simulink model "A"  (R2024b)
settings: Solver=VariableStepAuto  StartTime=0.0  StopTime=0.5  RelTol=1e-3
undefined symbols (not defined in the file): Ion, Lithium
libraries: spsSeriesRLCBranchLib x11, spsVoltageMeasurementLib x7, spsMosfetLib x6, spsCurrentMeasurementLib x4, spsPVArrayLib x2, spsDiodeLib x2, spsBatteryLib x2, slpidlib x2, spsTriangleGeneratorLib x2, spsBreakerLib x1, spspowerguiLib x1
settings Model: Creator=ASUS  LastModifiedBy=ASUS

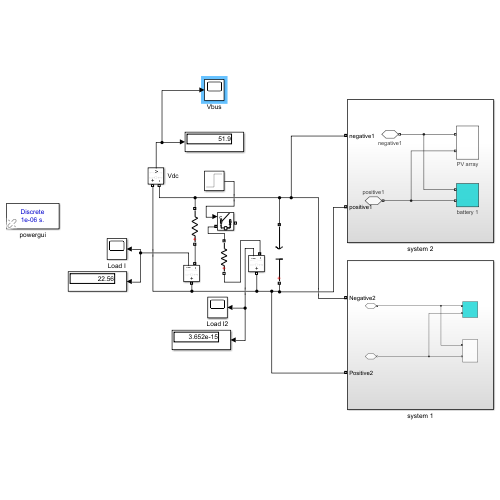
[thumbnail: Simulink's stored preview of the top-level diagram]
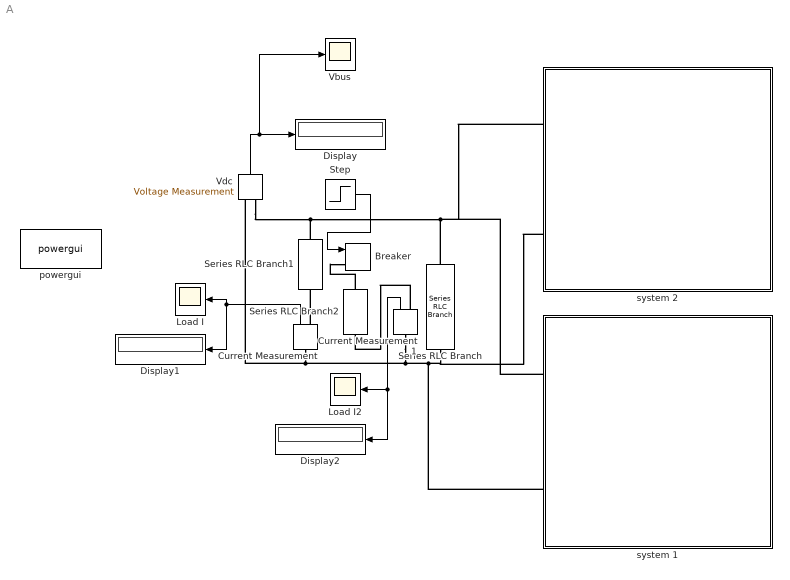
== system A ==
  Breaker : spsBreakerLib/Breaker  InitialState=0  SwitchingTimes="[1/60  5/60]"  External=on  BreakerResistance=0.01  SnubberResistance=1e6  SnubberCapacitance=inf  Measurements=None  MoreParameters=on  NoBreakLoop=off
  Current Measurement : spsCurrentMeasurementLib/Current Measurement  PhasorSimulation=off  OutputType=Complex  PSBequivalent=0
  Current Measurement1 : spsCurrentMeasurementLib/Current Measurement  PhasorSimulation=off  OutputType=Complex  PSBequivalent=0
  Display : Display
  Display1 : Display
  Display2 : Display
  Load I : Scope
  Load I2 : Scope
  Series RLC Branch : spsSeriesRLCBranchLib/Series RLC Branch  LConnTagsString=__new0  RConnTagsString=__new0  BranchType=C  Resistance=1  Inductance=1e-3  SetiL0=off  InitialCurrent=0  Capacitance=4700e-6  Setx0=off  InitialVoltage=0  Measurements=None
  Series RLC Branch1 : spsSeriesRLCBranchLib/Series RLC Branch  LConnTagsString=__new0  RConnTagsString=__new0  BranchType=R  Resistance=2.3  Inductance=1e-3  SetiL0=off  InitialCurrent=0  Capacitance=4700e-6  Setx0=off  InitialVoltage=0  Measurements=None
  Series RLC Branch2 : spsSeriesRLCBranchLib/Series RLC Branch  LConnTagsString=__new0  RConnTagsString=__new0  BranchType=R  Resistance=2.3  Inductance=1e-3  SetiL0=off  InitialCurrent=0  Capacitance=4700e-6  Setx0=off  InitialVoltage=0  Measurements=None
  Step : Step  Time=0.2  SampleTime=0
  Vbus : Scope
  Vdc : spsVoltageMeasurementLib/Voltage Measurement  PhasorSimulation=off  OutputType=Complex  PSBequivalent=0
  powergui : spspowerguiLib/powergui  Priority=1  SimulationMode=Discrete  SampleTime=1e-6  frequency=60  Iterations=50  frequencyindice=0  Pbase=100e6  ErrMax=1e-4  UnitsV=kV  UnitsW=MW  buscounter=0  FunctionMessages=off  echomessages=off  EnableUseOfTLC=off  CurrentSourceSwitches=off  DisableSnubberDevices=off  DisableRonSwitches=off  DisableVfSwitches=off  DisplayEquations=off  AutomaticDiscreteSolvers=off  SolverType=Tustin/Backward Euler (TBE)  Interpol=off  ExternalGateDelay=off  methode=off  Ts=100  x0status=blocks  SPID=on  SwTol=0  HookPort=off  NonlinearTolerance=1e-4  nMaxIteration=100  ContinueOnMaxIteration=off  RestoreLinks=warning  ResistiveCurrentMeasurement=off  Frange=[0:2:500]  Ylog=off  Xlog=on  ShowGrid=off  save=off  variable=ZData  structure=0  ZoomFFT=off  StartTime=0.0  cycles=1  DisplayStyle=1  fundamental=60  FreqAxis=off  MaxFrequency=1000  frequencyindicesteady=1  RmsSteady=1  display=off
  system 1 : Subsystem
  system 2 : Subsystem
  wires:
  Vdc/1 -> Vbus/1, Display/1
  Step/1 -> Breaker/1
  Current Measurement/1 -> Load I/1, Display1/1
  Current Measurement1/1 -> Display2/1, Load I2/1
  connections:
  system 2/LConn2 -- Series RLC Branch/LConn1 -- system 1/LConn2 -- Current Measurement1/LConn1 -- Current Measurement/LConn1 -- Vdc/LConn1
  Vdc/LConn2 -- Series RLC Branch1/RConn1 -- system 2/LConn1 -- system 1/LConn1 -- Series RLC Branch/RConn1
  Series RLC Branch2/RConn1 -- Breaker/LConn1
  Current Measurement/RConn1 -- Series RLC Branch1/LConn1
  Current Measurement1/RConn1 -- Series RLC Branch2/LConn1

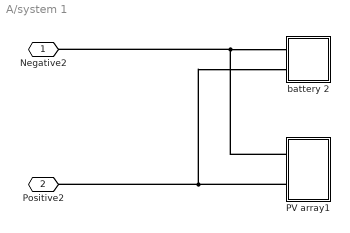
== system A/system 1 ==
  PV array1 : Subsystem
  battery 2 : Subsystem
  Negative2 : PMIOPort  Side=Left
  Positive2 : PMIOPort  Port=2  Side=Left
  connections:
  PV array1/LConn2 -- Positive2/RConn1 -- battery 2/LConn2
  PV array1/LConn1 -- Negative2/RConn1 -- battery 2/LConn1

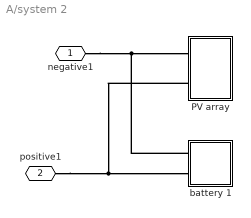
== system A/system 2 ==
  PV array : Subsystem
  battery 1 : Subsystem
  negative1 : PMIOPort  Side=Left
  positive1 : PMIOPort  Port=2  Side=Left
  connections:
  PV array/LConn2 -- positive1/RConn1 -- battery 1/LConn2
  battery 1/LConn1 -- negative1/RConn1 -- PV array/LConn1

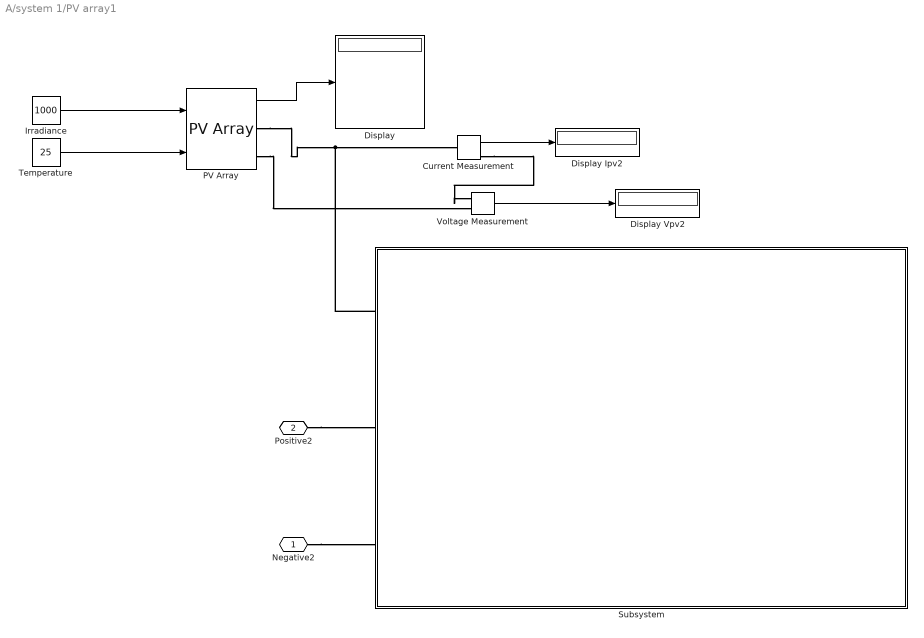
== system A/system 1/PV array1 ==
  Current Measurement : spsCurrentMeasurementLib/Current Measurement  PhasorSimulation=off  OutputType=Complex  PSBequivalent=0
  Display : Display
  Display Ipv2 : Display
  Display Vpv2 : Display
  Irradiance : Constant  Value=1000
  PV Array : spsPVArrayLib/PV Array  Npar=5  Nser=1  PlotType=array @ 1000 W/m2 & specified temperatures  S_vec="[ 1000  500  100 ]"  Temp_C_vec="[ 45 25  ]"  ModuleName=Kyocera Solar KC200GT  PlotWhenSelected=off  Pm=200.143  Ncell=54  Voc=32.9  Isc=8.21  Vm=26.3  Im=7.61  beta_Voc_pc=-0.355  alpha_Isc_pc=0.06  beta_Voc=-0.11679  alpha_Isc=0.004926  IL=8.2288  I0=2.3234e-10  nI=0.97734  Rsh=150.6844  Rs=0.34484  RobustModel=off  RobustCellTemperature=313.3991  BAL=off  Tc=1e-6  Tfilter=5e-5
  Subsystem : Subsystem
  Temperature : Constant  Value=25
  Voltage Measurement : spsVoltageMeasurementLib/Voltage Measurement  PhasorSimulation=off  OutputType=Complex  PSBequivalent=0
  Negative2 : PMIOPort  Side=Left
  Positive2 : PMIOPort  Port=2  Side=Left
  wires:
  Current Measurement/1 -> Display Ipv2/1
  Irradiance/1 -> PV Array/1
  Voltage Measurement/1 -> Display Vpv2/1
  PV Array/1 -> Display/1
  Temperature/1 -> PV Array/2
  connections:
  PV Array/RConn1 -- Subsystem/LConn1 -- Current Measurement/LConn1
  PV Array/RConn2 -- Voltage Measurement/LConn2
  Current Measurement/RConn1 -- Voltage Measurement/LConn1
  Negative2/RConn1 -- Subsystem/LConn3
  Positive2/RConn1 -- Subsystem/LConn2

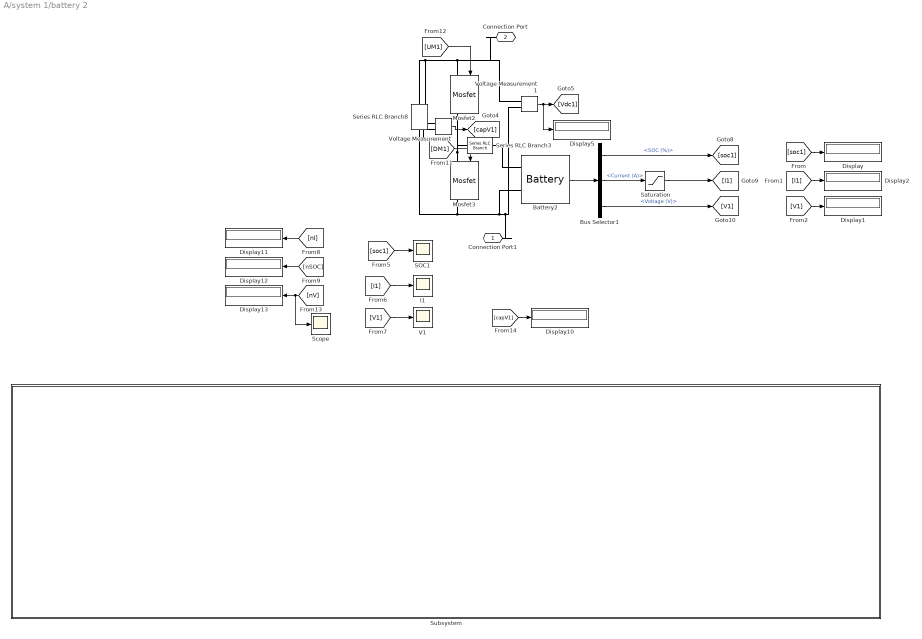
== system A/system 1/battery 2 ==
  Battery2 : spsBatteryLib/Battery  BatType=Lithium-Ion  NomV=50  NomQ=5  SOC=60  Batt_Tr=30  PresetModel=on  MaxQ=5  MinV=37.5  FullV=58.1994  Dis_rate=2.1739  R=0.1  Normal_OP=4.5217  expZone="[54.0193     0.245652]"
  Bus Selector1 : BusSelector  OutputSignals=SOC (%),Current (A),Voltage (V)
  Display{,1..2,5,10..13} (8 alike) : Display
  I1 : Scope
  Mosfet2 : spsMosfetLib/Mosfet  Ron=0.1  Lon=0  Rd=0.01  Vfd=0  IC=0  Rs=1e6  Cs=inf  Measurements=on
  Mosfet3 : spsMosfetLib/Mosfet  Ron=0.1  Lon=0  Rd=0.01  Vfd=0  IC=0  Rs=1e6  Cs=inf  Measurements=on
  SOC1 : Scope
  Saturation : Saturate  UpperLimit=31.5  LowerLimit=-31.5
  Scope : Scope
  Series RLC Branch3 : spsSeriesRLCBranchLib/Series RLC Branch  LConnTagsString=__new0  RConnTagsString=__new0  BranchType=L  Resistance=1  Inductance=500e-6  SetiL0=off  InitialCurrent=0  Capacitance=1e-6  Setx0=off  InitialVoltage=0  Measurements=None
  Series RLC Branch8 : spsSeriesRLCBranchLib/Series RLC Branch  LConnTagsString=__new0  RConnTagsString=__new0  BranchType=RC  Resistance=1  Inductance=1e-3  SetiL0=off  InitialCurrent=0  Capacitance=1500e-6  Setx0=off  InitialVoltage=0  Measurements=None
  Subsystem : Subsystem
  V1 : Scope
  Voltage Measurement : spsVoltageMeasurementLib/Voltage Measurement  PhasorSimulation=off  OutputType=Complex  PSBequivalent=0
  Voltage Measurement1 : spsVoltageMeasurementLib/Voltage Measurement  PhasorSimulation=off  OutputType=Complex  PSBequivalent=0
  Connection Port1 : PMIOPort  Side=Left
  Connection Port : PMIOPort  Port=2  Side=Left
  wires:
  [soc1] -> Display/1
  Voltage Measurement/1 -> [capV1]
  [nSOC] -> Display12/1
  [V1] -> V1/1
  [nI] -> Display11/1
  Bus Selector1/3 -> [V1]  "<Voltage (V)>"
  [UM1] -> Mosfet2/1
  Battery2/1 -> Bus Selector1/1
  [I1] -> Display2/1
  [soc1] -> SOC1/1
  [nV] -> Display13/1, Scope/1
  Bus Selector1/1 -> [soc1]  "<SOC (%)>"
  [I1] -> I1/1
  [capV1] -> Display10/1
  [V1] -> Display1/1
  [DM1] -> Mosfet3/1
  Voltage Measurement1/1 -> [Vdc1], Display5/1
  Saturation/1 -> [I1]
  Bus Selector1/2 -> Saturation/1  "<Current (A)>"
  connections:
  Mosfet3/LConn1 -- Series RLC Branch3/RConn1 -- Mosfet2/RConn1
  Voltage Measurement1/LConn2 -- Connection Port1/RConn1 -- Mosfet3/RConn1 -- Voltage Measurement/LConn2 -- Series RLC Branch8/RConn1 -- Battery2/LConn2
  Voltage Measurement/LConn1 -- Connection Port/RConn1 -- Voltage Measurement1/LConn1 -- Mosfet2/LConn1 -- Series RLC Branch8/LConn1
  Battery2/LConn1 -- Series RLC Branch3/LConn1

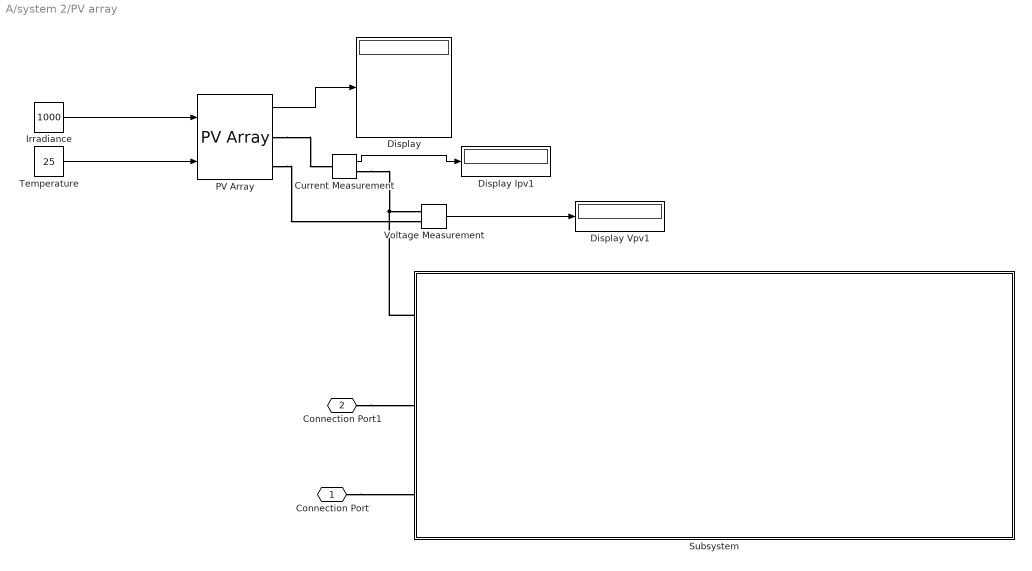
== system A/system 2/PV array ==
  Current Measurement : spsCurrentMeasurementLib/Current Measurement  PhasorSimulation=off  OutputType=Complex  PSBequivalent=0
  Display : Display
  Display Ipv1 : Display
  Display Vpv1 : Display
  Irradiance : Constant  Value=1000
  PV Array : spsPVArrayLib/PV Array  Npar=5  Nser=1  PlotType=array @ 1000 W/m2 & specified temperatures  S_vec="[ 1000  500  100 ]"  Temp_C_vec="[ 45 25  ]"  ModuleName=Kyocera Solar KC200GT  PlotWhenSelected=off  Pm=200.143  Ncell=54  Voc=32.9  Isc=8.21  Vm=26.3  Im=7.61  beta_Voc_pc=-0.355  alpha_Isc_pc=0.06  beta_Voc=-0.11679  alpha_Isc=0.004926  IL=8.2288  I0=2.3234e-10  nI=0.97734  Rsh=150.6844  Rs=0.34484  RobustModel=off  RobustCellTemperature=313.3991  BAL=off  Tc=1e-6  Tfilter=5e-5
  Subsystem : Subsystem
  Temperature : Constant  Value=25
  Voltage Measurement : spsVoltageMeasurementLib/Voltage Measurement  PhasorSimulation=off  OutputType=Complex  PSBequivalent=0
  Connection Port : PMIOPort  Side=Left
  Connection Port1 : PMIOPort  Port=2  Side=Left
  wires:
  Temperature/1 -> PV Array/2
  PV Array/1 -> Display/1
  Voltage Measurement/1 -> Display Vpv1/1
  Irradiance/1 -> PV Array/1
  Current Measurement/1 -> Display Ipv1/1
  connections:
  Current Measurement/RConn1 -- Subsystem/LConn1 -- Voltage Measurement/LConn1
  PV Array/RConn2 -- Voltage Measurement/LConn2
  PV Array/RConn1 -- Current Measurement/LConn1
  Connection Port1/RConn1 -- Subsystem/LConn2
  Connection Port/RConn1 -- Subsystem/LConn3

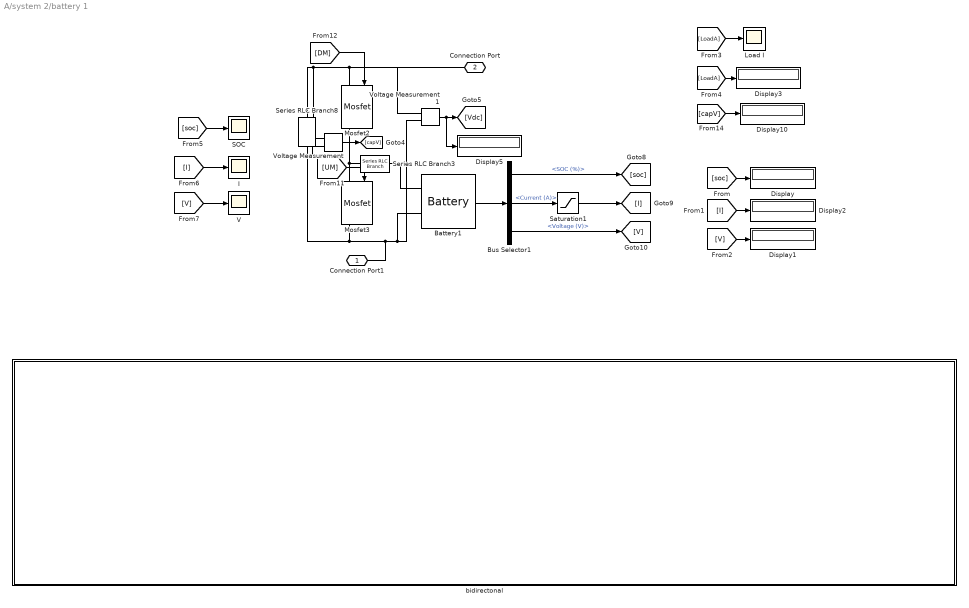
== system A/system 2/battery 1 ==
  Battery1 : spsBatteryLib/Battery  BatType=Lithium-Ion  NomV=48  NomQ=100  SOC=80  Batt_Tr=30  PresetModel=on  MaxQ=100  MinV=36  FullV=55.8714  Dis_rate=43.4783  R=0.0048  Normal_OP=90.4348  expZone="[51.8585      4.91304]"
  Bus Selector1 : BusSelector  OutputSignals=SOC (%),Current (A),Voltage (V)
  Display{,1..3,5,10} (6 alike) : Display
  I : Scope
  Load I : Scope
  Mosfet2 : spsMosfetLib/Mosfet  Ron=0.1  Lon=0  Rd=0.01  Vfd=0  IC=0  Rs=1e6  Cs=inf  Measurements=on
  Mosfet3 : spsMosfetLib/Mosfet  Ron=0.1  Lon=0  Rd=0.01  Vfd=0  IC=0  Rs=1e6  Cs=inf  Measurements=on
  SOC : Scope
  Saturation1 : Saturate  UpperLimit=31.5  LowerLimit=-31.5
  Series RLC Branch3 : spsSeriesRLCBranchLib/Series RLC Branch  LConnTagsString=__new0  RConnTagsString=__new0  BranchType=L  Resistance=1  Inductance=500e-6  SetiL0=off  InitialCurrent=0  Capacitance=1e-6  Setx0=off  InitialVoltage=0  Measurements=None
  Series RLC Branch8 : spsSeriesRLCBranchLib/Series RLC Branch  LConnTagsString=__new0  RConnTagsString=__new0  BranchType=RC  Resistance=1  Inductance=1e-3  SetiL0=off  InitialCurrent=0  Capacitance=1500e-6  Setx0=off  InitialVoltage=0  Measurements=None
  V : Scope
  Voltage Measurement : spsVoltageMeasurementLib/Voltage Measurement  PhasorSimulation=off  OutputType=Complex  PSBequivalent=0
  Voltage Measurement1 : spsVoltageMeasurementLib/Voltage Measurement  PhasorSimulation=off  OutputType=Complex  PSBequivalent=0
  bidirectonal : Subsystem
  Connection Port1 : PMIOPort  Side=Left
  Connection Port : PMIOPort  Port=2  Side=Left
  wires:
  Voltage Measurement1/1 -> Display5/1, [Vdc]
  [UM] -> Mosfet3/1
  [V] -> Display1/1
  [capV] -> Display10/1
  [I] -> I/1
  Bus Selector1/1 -> [soc]  "<SOC (%)>"
  [soc] -> SOC/1
  [I] -> Display2/1
  Battery1/1 -> Bus Selector1/1
  [DM] -> Mosfet2/1
  Bus Selector1/3 -> [V]  "<Voltage (V)>"
  [LoadA] -> Load I/1
  [V] -> V/1
  Voltage Measurement/1 -> [capV]
  [LoadA] -> Display3/1
  [soc] -> Display/1
  Bus Selector1/2 -> Saturation1/1  "<Current (A)>"
  Saturation1/1 -> [I]
  connections:
  Battery1/LConn1 -- Series RLC Branch3/LConn1
  Series RLC Branch8/LConn1 -- Voltage Measurement1/LConn1 -- Connection Port/RConn1 -- Mosfet2/LConn1 -- Voltage Measurement/LConn1
  Battery1/LConn2 -- Connection Port1/RConn1 -- Series RLC Branch8/RConn1 -- Voltage Measurement/LConn2 -- Mosfet3/RConn1 -- Voltage Measurement1/LConn2
  Mosfet2/RConn1 -- Series RLC Branch3/RConn1 -- Mosfet3/LConn1

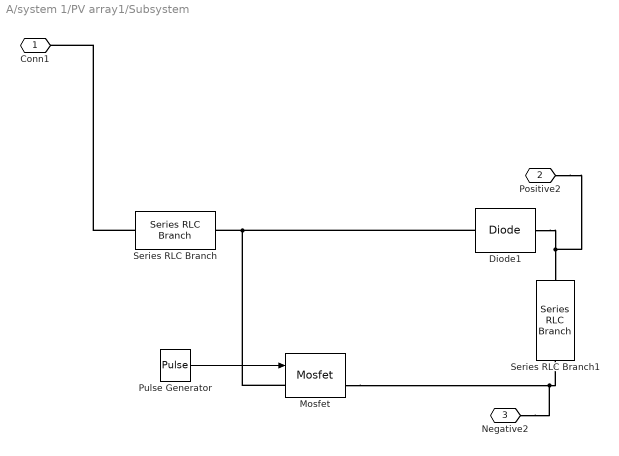
== system A/system 1/PV array1/Subsystem ==
  Diode1 : spsDiodeLib/Diode  Ron=0.001  Lon=0  Vf=0.8  IC=0  UseSnubber=0  Rs=500  Cs=250e-9  Measurements=off
  Mosfet : spsMosfetLib/Mosfet  Ron=0.001  Lon=0  Rd=0.01  Vfd=0.8  IC=0  Rs=1e4  Cs=inf  Measurements=on
  Pulse Generator : DiscretePulseGenerator  PulseType=Time based  Period=0.0001  PulseWidth=50
  Series RLC Branch : spsSeriesRLCBranchLib/Series RLC Branch  LConnTagsString=__new0  RConnTagsString=__new0  BranchType=L  Resistance=1  Inductance=5e-4  SetiL0=off  InitialCurrent=0  Capacitance=1e-6  Setx0=off  InitialVoltage=0  Measurements=None
  Series RLC Branch1 : spsSeriesRLCBranchLib/Series RLC Branch  LConnTagsString=__new0  RConnTagsString=__new0  BranchType=C  Resistance=1  Inductance=1e-3  SetiL0=off  InitialCurrent=0  Capacitance=470e-6  Setx0=off  InitialVoltage=0  Measurements=None
  Conn1 : PMIOPort  Side=Left
  Positive2 : PMIOPort  Port=2  Side=Left
  Negative2 : PMIOPort  Port=3  Side=Left
  wires:
  Pulse Generator/1 -> Mosfet/1
  connections:
  Diode1/LConn1 -- Mosfet/LConn1 -- Series RLC Branch/RConn1
  Mosfet/RConn1 -- Negative2/RConn1 -- Series RLC Branch1/RConn1
  Diode1/RConn1 -- Positive2/RConn1 -- Series RLC Branch1/LConn1
  Series RLC Branch/LConn1 -- Conn1/RConn1

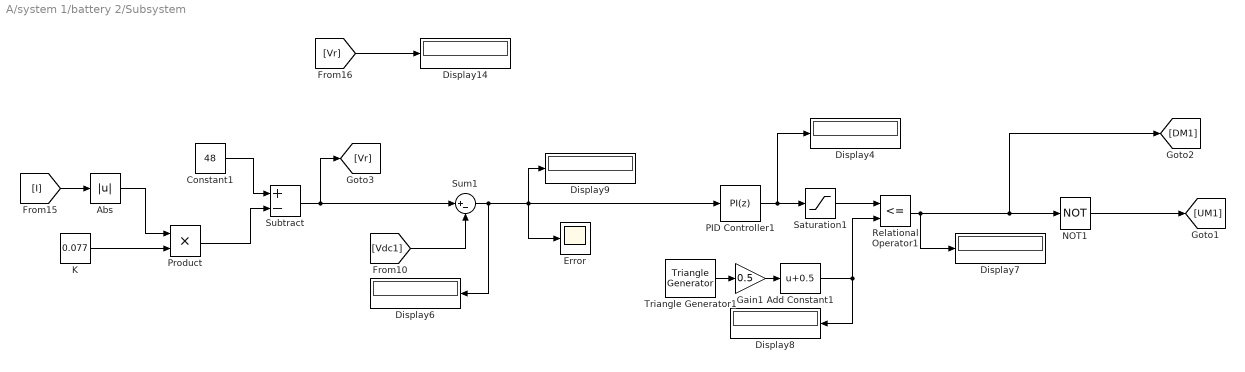
== system A/system 1/battery 2/Subsystem ==
  Abs : Abs  SaturateOnIntegerOverflow=off
  Add Constant1 : Bias  Bias=0.5  SaturateOnIntegerOverflow=off
  Constant1 : Constant  Value=48
  Display{4,6..9,14} (6 alike) : Display
  Error : Scope
  Gain1 : Gain  Gain=0.5
  K : Constant  Value=0.077
  NOT1 : Logic  Operator=NOT  IconShape=distinctive  AllPortsSameDT=off  OutDataTypeStr=boolean
  PID Controller1 : slpidlib/PID Controller  Controller=PI  Form=Parallel  TimeDomain=Discrete-time  UseExternalTs=off  SampleTime=-1  IntegratorMethod=Forward Euler  FilterMethod=Forward Euler  ControllerParametersSource=internal  P=0.08  I=10  UseKiTs=off  D=0  UseExternalDerivativeSource=off  N=100  UseFilter=on  TunerSelectOption=Transfer Function Based (PID Tuner App)  ZeroCross=off  InitialConditionSource=internal  InitialConditionForIntegrator=0  InitialConditionForFilter=0  DifferentiatorICPrevScaledInput=0  ExternalReset=none  TrackingMode=off  Kt=1  LimitOutput=on  SatLimitsSource=internal  UpperSaturationLimit=1  LowerSaturationLimit=-1  LinearizeAsGain=on  AntiWindupMode=back-calculation  Kb=1  LimitIntegrator=off  UpperIntegratorSaturationLimit=inf  LowerIntegratorSaturationLimit=-inf  POutMin=[]  POutMax=[]  IOutMin=[]  IOutMax=[]  DOutMin=[]  DOutMax=[]  NOutMin=[]  NOutMax=[]  SumOutMin=[]  SumOutMax=[]  SaturationOutMin=[]  SaturationOutMax=[]  PParamMin=[]  PParamMax=[]  IParamMin=[]  IParamMax=[]  DParamMin=[]  DParamMax=[]  NParamMin=[]  NParamMax=[]  KbParamMin=[]  KbParamMax=[]  KtParamMin=[]  KtParamMax=[]  KbOutMin=[]  KbOutMax=[]  KtOutMin=[]  KtOutMax=[]  IntegratorOutMin=[]  IntegratorOutMax=[]  FilterOutMin=[]  FilterOutMax=[]  SumI1OutMin=[]  SumI1OutMax=[]  SumI2OutMin=[]  SumI2OutMax=[]  SumI3OutMin=[]  SumI3OutMax=[]  SumI4OutMin=[]  SumI4OutMax=[]  SumDOutMin=[]  SumDOutMax=[]  DifferentiatorOutMin=[]  DifferentiatorOutMax=[]  FilterDiffOutCoefMin=[]  FilterDiffOutCoefMax=[]  ReciprocalOutMin=[]  ReciprocalOutMax=[]  SumDenOutMin=[]  SumDenOutMax=[]  SumNumOutMin=[]  SumNumOutMax=[]  DivideOutMin=[]  DivideOutMax=[]  UdiffTsProdOutMin=[]  UdiffTsProdOutMax=[]  NTsProdOutMin=[]  NTsProdOutMax=[]  UintegralTsProdOutMin=[]  UintegralTsProdOutMax=[]  UngainTsProdOutMin=[]  UngainTsProdOutMax=[]  ClampingZeroOutDataTypeStr=Inherit: Inherit via back propagation  ClampingZeroOutMin=[]  ClampingZeroOutMax=[]  FilterDenConstantOutDataTypeStr=Inherit: Inherit via back propagation  FilterDenConstantOutMin=[]  FilterDenConstantOutMax=[]  PCopyOutDataTypeStr=Inherit: Inherit via back propagation  PCopyOutMin=[]  PCopyOutMax=[]  NCopyOutDataTypeStr=Inherit: Inherit via back propagation  NCopyOutMin=[]  NCopyOutMax=[]  IntegratorContinuousStateAttributes=''  IntegratorStateMustResolveToSignalObject=off  IntegratorRTWStateStorageClass=Auto  FilterContinuousStateAttributes=''  FilterStateMustResolveToSignalObject=off  FilterRTWStateStorageClass=Auto  ParallelPVariant=InternalParameters  IdealPVariant=Disabled  IVariant=InternalParameters  DVariant=Disabled  IntegratorVariant=Discrete  SatVariant=Enabled  AWVariant=BackCalculation  PCopyVariant=Disabled  TRVariant=Disabled  FdbkBlocksVariant=Forward  IdealPFdbkVariant=Disabled  SatFdbkVariant=Disabled  DerivativeFilterVariant=Disabled  NVariant=Disabled  NCopyVariant=Disabled_SignalSpec  FilterICVariant=Disabled  IntegratorICVariant=InternalICs  ExternalResetVariant=Disabled  TRSumVariant=Passthrough  SumFdbkVariant=Disabled  SumVariant=Sum_PI  TsampFilterVariant=InternalTs  TsampNgainVariant=Passthrough  TsampIntegralVariant=Disabled_SignalSpec  ExternalSaturationOutDataTypeStr=Inherit: Same as second input  DerivativeSourceVariant=Disabled  PreIntVariant=InternalPreInt
  Product : Product
  Relational Operator1 : RelationalOperator  Operator=<=  OutDataTypeStr=boolean  RndMeth=Simplest  InputSameDT=off
  Saturation1 : Saturate  UpperLimit=0.95  LowerLimit=0.5
  Subtract : Sum  Inputs=+-
  Sum1 : Sum  Inputs=|+-
  Triangle Generator1 : spsTriangleGeneratorLib/Triangle Generator  Freq=10000  Phase=0  Ts=1e-6
  wires:
  K/1 -> Product/2
  Abs/1 -> Product/1
  PID Controller1/1 -> Saturation1/1, Display4/1
  Saturation1/1 -> Relational Operator1/1
  [Vr] -> Display14/1
  Add Constant1/1 -> Relational Operator1/2, Display8/1
  Constant1/1 -> Subtract/1
  NOT1/1 -> [UM1]
  [I] -> Abs/1
  Relational Operator1/1 -> Display7/1, [DM1], NOT1/1
  [Vdc1] -> Sum1/2
  Gain1/1 -> Add Constant1/1
  Sum1/1 -> Display6/1, Error/1, PID Controller1/1, Display9/1
  Subtract/1 -> [Vr], Sum1/1
  Product/1 -> Subtract/2
  Triangle Generator1/1 -> Gain1/1

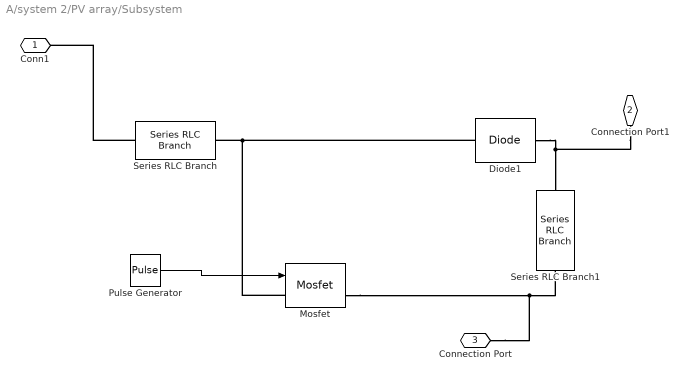
== system A/system 2/PV array/Subsystem ==
  Diode1 : spsDiodeLib/Diode  Ron=0.001  Lon=0  Vf=0.8  IC=0  UseSnubber=0  Rs=500  Cs=250e-9  Measurements=off
  Mosfet : spsMosfetLib/Mosfet  Ron=0.001  Lon=0  Rd=0.01  Vfd=0.8  IC=0  Rs=1e4  Cs=inf  Measurements=on
  Pulse Generator : DiscretePulseGenerator  PulseType=Time based  Period=0.0001  PulseWidth=50
  Series RLC Branch : spsSeriesRLCBranchLib/Series RLC Branch  LConnTagsString=__new0  RConnTagsString=__new0  BranchType=L  Resistance=1  Inductance=5e-4  SetiL0=off  InitialCurrent=0  Capacitance=1e-6  Setx0=off  InitialVoltage=0  Measurements=None
  Series RLC Branch1 : spsSeriesRLCBranchLib/Series RLC Branch  LConnTagsString=__new0  RConnTagsString=__new0  BranchType=C  Resistance=1  Inductance=1e-3  SetiL0=off  InitialCurrent=0  Capacitance=470e-6  Setx0=off  InitialVoltage=0  Measurements=None
  Conn1 : PMIOPort  Side=Left
  Connection Port1 : PMIOPort  Port=2  Side=Left
  Connection Port : PMIOPort  Port=3  Side=Left
  wires:
  Pulse Generator/1 -> Mosfet/1
  connections:
  Diode1/RConn1 -- Connection Port1/RConn1 -- Series RLC Branch1/LConn1
  Diode1/LConn1 -- Mosfet/LConn1 -- Series RLC Branch/RConn1
  Mosfet/RConn1 -- Connection Port/RConn1 -- Series RLC Branch1/RConn1
  Series RLC Branch/LConn1 -- Conn1/RConn1

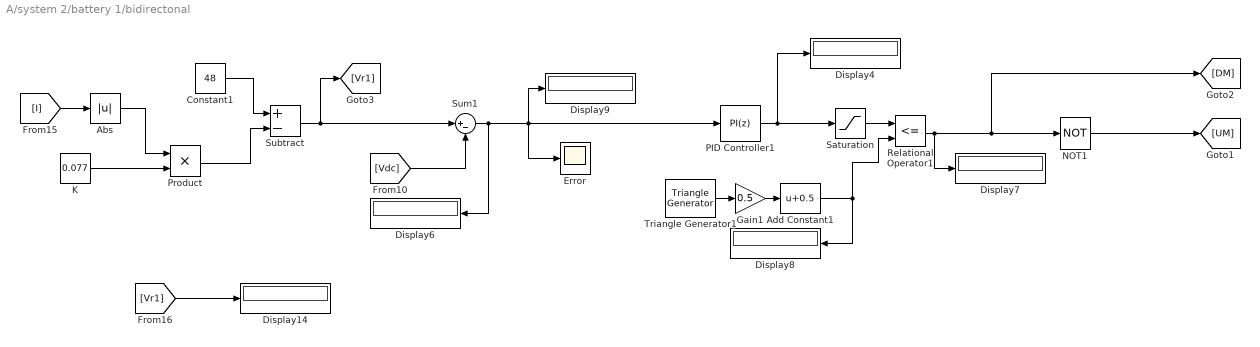
== system A/system 2/battery 1/bidirectonal ==
  Abs : Abs  SaturateOnIntegerOverflow=off
  Add Constant1 : Bias  Bias=0.5  SaturateOnIntegerOverflow=off
  Constant1 : Constant  Value=48
  Display{4,6..9,14} (6 alike) : Display
  Error : Scope
  Gain1 : Gain  Gain=0.5
  K : Constant  Value=0.077
  NOT1 : Logic  Operator=NOT  IconShape=distinctive  AllPortsSameDT=off  OutDataTypeStr=boolean
  PID Controller1 : slpidlib/PID Controller  Controller=PI  Form=Parallel  TimeDomain=Discrete-time  UseExternalTs=off  SampleTime=-1  IntegratorMethod=Forward Euler  FilterMethod=Forward Euler  ControllerParametersSource=internal  P=0.08  I=10  UseKiTs=off  D=0  UseExternalDerivativeSource=off  N=100  UseFilter=on  TunerSelectOption=Transfer Function Based (PID Tuner App)  ZeroCross=off  InitialConditionSource=internal  InitialConditionForIntegrator=0  InitialConditionForFilter=0  DifferentiatorICPrevScaledInput=0  ExternalReset=none  TrackingMode=off  Kt=1  LimitOutput=on  SatLimitsSource=internal  UpperSaturationLimit=1  LowerSaturationLimit=-1  LinearizeAsGain=on  AntiWindupMode=back-calculation  Kb=1  LimitIntegrator=off  UpperIntegratorSaturationLimit=inf  LowerIntegratorSaturationLimit=-inf  POutMin=[]  POutMax=[]  IOutMin=[]  IOutMax=[]  DOutMin=[]  DOutMax=[]  NOutMin=[]  NOutMax=[]  SumOutMin=[]  SumOutMax=[]  SaturationOutMin=[]  SaturationOutMax=[]  PParamMin=[]  PParamMax=[]  IParamMin=[]  IParamMax=[]  DParamMin=[]  DParamMax=[]  NParamMin=[]  NParamMax=[]  KbParamMin=[]  KbParamMax=[]  KtParamMin=[]  KtParamMax=[]  KbOutMin=[]  KbOutMax=[]  KtOutMin=[]  KtOutMax=[]  IntegratorOutMin=[]  IntegratorOutMax=[]  FilterOutMin=[]  FilterOutMax=[]  SumI1OutMin=[]  SumI1OutMax=[]  SumI2OutMin=[]  SumI2OutMax=[]  SumI3OutMin=[]  SumI3OutMax=[]  SumI4OutMin=[]  SumI4OutMax=[]  SumDOutMin=[]  SumDOutMax=[]  DifferentiatorOutMin=[]  DifferentiatorOutMax=[]  FilterDiffOutCoefMin=[]  FilterDiffOutCoefMax=[]  ReciprocalOutMin=[]  ReciprocalOutMax=[]  SumDenOutMin=[]  SumDenOutMax=[]  SumNumOutMin=[]  SumNumOutMax=[]  DivideOutMin=[]  DivideOutMax=[]  UdiffTsProdOutMin=[]  UdiffTsProdOutMax=[]  NTsProdOutMin=[]  NTsProdOutMax=[]  UintegralTsProdOutMin=[]  UintegralTsProdOutMax=[]  UngainTsProdOutMin=[]  UngainTsProdOutMax=[]  ClampingZeroOutDataTypeStr=Inherit: Inherit via back propagation  ClampingZeroOutMin=[]  ClampingZeroOutMax=[]  FilterDenConstantOutDataTypeStr=Inherit: Inherit via back propagation  FilterDenConstantOutMin=[]  FilterDenConstantOutMax=[]  PCopyOutDataTypeStr=Inherit: Inherit via back propagation  PCopyOutMin=[]  PCopyOutMax=[]  NCopyOutDataTypeStr=Inherit: Inherit via back propagation  NCopyOutMin=[]  NCopyOutMax=[]  IntegratorContinuousStateAttributes=''  IntegratorStateMustResolveToSignalObject=off  IntegratorRTWStateStorageClass=Auto  FilterContinuousStateAttributes=''  FilterStateMustResolveToSignalObject=off  FilterRTWStateStorageClass=Auto  ParallelPVariant=InternalParameters  IdealPVariant=Disabled  IVariant=InternalParameters  DVariant=Disabled  IntegratorVariant=Discrete  SatVariant=Enabled  AWVariant=BackCalculation  PCopyVariant=Disabled  TRVariant=Disabled  FdbkBlocksVariant=Forward  IdealPFdbkVariant=Disabled  SatFdbkVariant=Disabled  DerivativeFilterVariant=Disabled  NVariant=Disabled  NCopyVariant=Disabled_SignalSpec  FilterICVariant=Disabled  IntegratorICVariant=InternalICs  ExternalResetVariant=Disabled  TRSumVariant=Passthrough  SumFdbkVariant=Disabled  SumVariant=Sum_PI  TsampFilterVariant=InternalTs  TsampNgainVariant=Passthrough  TsampIntegralVariant=Disabled_SignalSpec  ExternalSaturationOutDataTypeStr=Inherit: Same as second input  DerivativeSourceVariant=Disabled  PreIntVariant=InternalPreInt
  Product : Product
  Relational Operator1 : RelationalOperator  Operator=<=  OutDataTypeStr=boolean  RndMeth=Simplest  InputSameDT=off
  Saturation : Saturate  UpperLimit=0.95  LowerLimit=0.05
  Subtract : Sum  Inputs=+-
  Sum1 : Sum  Inputs=|+-
  Triangle Generator1 : spsTriangleGeneratorLib/Triangle Generator  Freq=10000  Phase=0  Ts=1e-6
  wires:
  Sum1/1 -> Display9/1, PID Controller1/1, Error/1, Display6/1
  K/1 -> Product/2
  Product/1 -> Subtract/2
  Subtract/1 -> Sum1/1, [Vr1]
  Constant1/1 -> Subtract/1
  Relational Operator1/1 -> [DM], NOT1/1, Display7/1
  [Vdc] -> Sum1/2
  Add Constant1/1 -> Display8/1, Relational Operator1/2
  Saturation/1 -> Relational Operator1/1
  PID Controller1/1 -> Saturation/1, Display4/1
  [Vr1] -> Display14/1
  NOT1/1 -> [UM]
  [I] -> Abs/1
  Gain1/1 -> Add Constant1/1
  Triangle Generator1/1 -> Gain1/1
  Abs/1 -> Product/1
